simulink model "RM3old"  (R2018b)
settings: Solver=ode4  StartTime=0  StopTime=72.5  FixedStep=0.001  MaxStep=0.001  RelTol=1e-3  EnableMultiTasking=on
undefined symbols (not defined in the file or in its folder): body, constraint, pto
libraries: WECSim_Lib x5
settings Model: Creator=mlawson  LastModifiedBy=David
settings SolverCC: ZeroCrossControl=DisableAll  AlgebraicLoopSolver=LineSearch  AutoInsertRateTranBlk=on
settings DataIOCC: SaveFormat=Array  SaveOutput=off  SaveTime=off
settings OptimizationCC: LifeSpan=inf  SimCompilerOptimization=on
settings DebuggingCC: UnderspecifiedInitializationDetection=Classic  MergeDetectMultiDrivingBlocksExec=none  SolverPrmCheckMsg=warning  AllowSymbolicDim=off  StateNameClashWarn=warning  SFUnexpectedBacktrackingDiag=warning  SFNoUnconditionalDefaultTransitionDiag=warning  SFExecutionAtInitializationDiag=none
settings HardwareCC: ProdBitPerPointer=32  ProdBitPerSizeT=32  ProdBitPerPtrDiffT=32  ProdLargestAtomicFloat=None  ProdIntDivRoundTo=Undefined  ProdEndianess=Unspecified  ProdWordSize=32  ProdHWDeviceType=32-bit Generic
settings ModelReferenceCC: PropagateSignalLabelsOutOfModel=off
settings SFSimCC: SimUseLocalCustomCode=off
settings RTWCC: RTWUseLocalCustomCode=off
settings CodeAppCC: StateflowObjectComments=on
settings GRTTargetCC: TargetLangStandard=C89/C90 (ANSI)  GeneratePreprocessorConditionals=Disable all
settings ConfigComp: CovMetricSettings=dw  CovHtmlReporting=on  CovSaveCumulativeToWorkspaceVar=on  CovSaveSingleToWorkspaceVar=on  CovExternalEMLEnable=off  CovSFcnEnable=off
settings SimscapeCC: SimscapeNormalizeSystem=off
settings ConfigurationSet: Description=SimMechanics 2G
settings ExplorerConfigSet: InternalSimMechanicsExplorerSettings="<ExplorerConfiguration><canonicalview>default</canonicalview><TilePanel><TileInfo><Tiles Columns=\"1\" Count=\"1\" Rows=\"1\"><Column Left=\"2\" Weight=\"1\"/><Column Left=\"1335\"/><Row Top=\"2\" Weight=\"1\"/><Row Top=\"911\"/><Tile Height=\"1\" Width=\"1\" X=\"0\" Y=\"0\"/></Tiles></TileInfo><SceneInfo><SceneViewer><BGColor><R>0.60000002384185791</R><G>0.60000002384185791</G><B>0.60000002384185791</B></BGColor><Camera><Position><X>365.37645888990272</X><Y>-369.82486814446582</Y><Z>359.64809521743916</Z></Position><Center><X>-6.7351450971904585</X><Y>2.2867358426280204</Y><Z>-12.463508769654169</Z></Center><Up><X>-0.40824829046386307</X><Y>0.40824829046386307</Y><Z>0.81649658092772615</Z></Up><Left>-57.820127362122818</Left><Right>57.820127362122818</Right><Bottom>-38.308817187253304</Bottom><Top>38.308817187253304</Top></Camera></SceneViewer></SceneInfo></TilePanel></ExplorerConfiguration>"

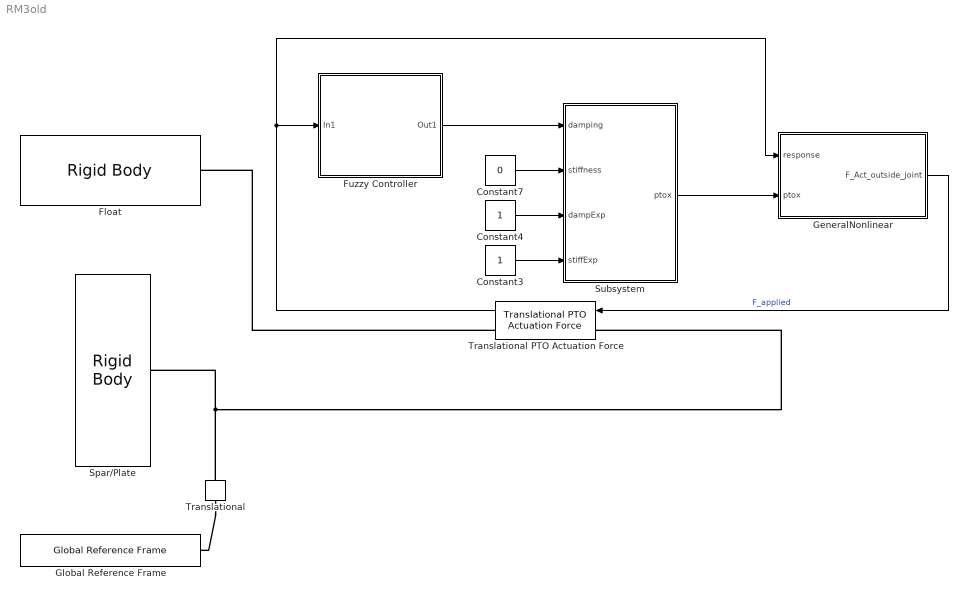
== system RM3old ==
  Constant3 : Constant
  Constant4 : Constant
  Constant7 : Constant  Value=0
  Float : WECSim_Lib/Body Elements/Rigid Body  body=body(1)
      settings: AttributesFormatString=%<body>  SourceProductName=WEC-Sim
  Fuzzy Controller : Subsystem
  GeneralNonlinear : Subsystem
  Global Reference Frame : WECSim_Lib/Frames/Global Reference Frame  waves=waves  simu=simu
      settings: SourceProductName=WEC-Sim
  Spar/Plate : WECSim_Lib/Body Elements/Rigid Body  body=body(2)
      settings: AttributesFormatString=%<body>  SourceProductName=WEC-Sim
  Subsystem : Subsystem
  Translational : WECSim_Lib/Constraints/Translational  constraint=constraint(1)
      settings: AttributesFormatString=%<constraint>  SourceProductName=WEC-Sim
  Translational PTO Actuation Force : WECSim_Lib/PTOs/Translational PTO Actuation Force  pto=pto(1)
      settings: AttributesFormatString=%<pto>  SourceProductName=WEC-Sim
  wires:
  GeneralNonlinear/1(F_Act_outside_joint) -> Translational PTO Actuation Force/1  "F_applied"
  Constant7/1 -> Subsystem/2(stiffness)
  Subsystem/1(ptox) -> GeneralNonlinear/2(ptox)
  Constant3/1 -> Subsystem/4(stiffExp)
  Translational PTO Actuation Force/1 -> GeneralNonlinear/1(response), Fuzzy Controller/1(In1)
  Constant4/1 -> Subsystem/3(dampExp)
  Fuzzy Controller/1(Out1) -> Subsystem/1(damping)
  connections:
  Translational/LConn1 -- Global Reference Frame/RConn1
  Translational/RConn1 -- Spar/Plate/RConn1 -- Translational PTO Actuation Force/LConn1
  Translational PTO Actuation Force/RConn1 -- Float/RConn1

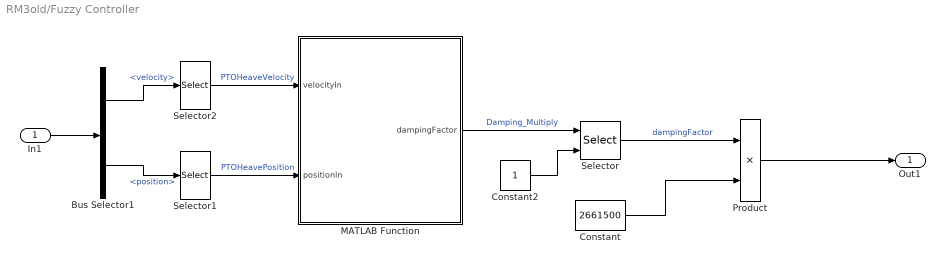
== system RM3old/Fuzzy Controller ==
  In1 : Inport
  Bus Selector1 : BusSelector  OutputSignals=velocity,position
  Constant : Constant  Value=2661500
  Constant2 : Constant
  MATLAB Function : MATLAB Function  TreatAsAtomicUnit=on  SystemSampleTime=0.01
  Product : Product
  Selector : Selector  InputPortWidth=2  IndexOptions=Index vector (port)  Indices=1  OutputSizes=1
  Selector1 : Selector  InputPortWidth=6  IndexOptions=Index vector (dialog)  Indices=3  OutputSizes=1
  Selector2 : Selector  InputPortWidth=6  IndexOptions=Index vector (dialog)  Indices=3  OutputSizes=1
  Out1 : Outport
  wires:
  Bus Selector1/2 -> Selector1/1  "<position>"
  Constant2/1 -> Selector/2
  Selector2/1 -> MATLAB Function/1(velocityIn)  "PTOHeaveVelocity"
  Bus Selector1/1 -> Selector2/1  "<velocity>"
  In1/1 -> Bus Selector1/1
  Selector1/1 -> MATLAB Function/2(positionIn)  "PTOHeavePosition"
  Selector/1 -> Product/1  "dampingFactor"
  Constant/1 -> Product/2
  MATLAB Function/1(dampingFactor) -> Selector/1  "Damping_Multiply"
  Product/1 -> Out1/1

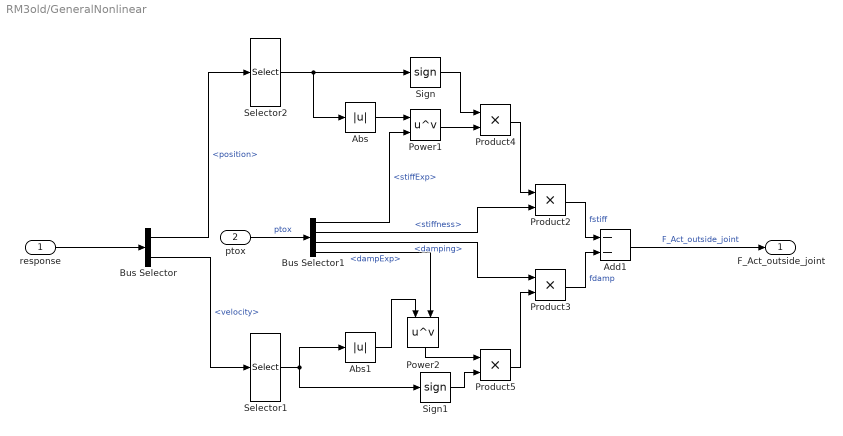
== system RM3old/GeneralNonlinear ==
  response : Inport
  ptox : Inport  Port=2
  Abs : Abs
  Abs1 : Abs
  Add1 : Sum  Inputs=--
  Bus Selector : BusSelector  OutputSignals=position,velocity
  Bus Selector1 : BusSelector  OutputSignals=stiffExp,stiffness,damping,dampExp
  Power1 : Math  Operator=pow  SaturateOnIntegerOverflow=on
  Power2 : Math  Operator=pow  SaturateOnIntegerOverflow=on
  Product2 : Product  Inputs=**
  Product3 : Product  Inputs=**
  Product4 : Product
  Product5 : Product
  Selector1 : Selector  InputPortWidth=6  IndexOptions=Index vector (dialog)  Indices=3  OutputSizes=1
  Selector2 : Selector  InputPortWidth=6  IndexOptions=Index vector (dialog)  Indices=3  OutputSizes=1
  Sign : Signum
  Sign1 : Signum
  F_Act_outside_joint : Outport
  wires:
  Power2/1 -> Product5/1
  Product5/1 -> Product3/2
  Sign/1 -> Product4/1
  Bus Selector1/3 -> Product3/1  "<damping>"
  Product2/1 -> Add1/1  "fstiff"
  response/1 -> Bus Selector/1
  Bus Selector1/1 -> Power1/2  "<stiffExp>"
  Bus Selector/2 -> Selector1/1  "<velocity>"
  Selector2/1 -> Sign/1, Abs/1
  Product4/1 -> Product2/1
  Add1/1 -> F_Act_outside_joint/1  "F_Act_outside_joint"
  Abs1/1 -> Power2/1
  Product3/1 -> Add1/2  "fdamp"
  Sign1/1 -> Product5/2
  Bus Selector1/2 -> Product2/2  "<stiffness>"
  Selector1/1 -> Abs1/1, Sign1/1
  Power1/1 -> Product4/2
  Bus Selector/1 -> Selector2/1  "<position>"
  Abs/1 -> Power1/1
  ptox/1 -> Bus Selector1/1  "ptox"
  Bus Selector1/4 -> Power2/2  "<dampExp>"

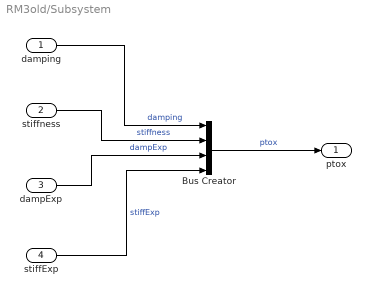
== system RM3old/Subsystem ==
  damping : Inport
  stiffness : Inport  Port=2
  dampExp : Inport  Port=3
  stiffExp : Inport  Port=4
  Bus Creator : BusCreator  Inputs=4
  ptox : Outport
  wires:
  stiffness/1 -> Bus Creator/2  "stiffness"
  stiffExp/1 -> Bus Creator/4  "stiffExp"
  Bus Creator/1 -> ptox/1  "ptox"
  damping/1 -> Bus Creator/1  "damping"
  dampExp/1 -> Bus Creator/3  "dampExp"

== matlab function RM3old/Fuzzy Controller/MATLAB Function ==
  data: velocityIn input; positionIn input; dampingFactor output size=[1 2]
function dampingFactor =...
    fuzzyLogicController(velocityIn, positionIn)
% Function to create and evaluate a fuzzy logic controller
% which implements a protection system for RM3 to limit relative movement
% between the float and spar, shedding power in the event of too-high wave conditions. The
% PTO implements an optimally linear damped control when within the travel limits,
% and applies a multiplication factor to the damping if the float is close
% to traveling out of bounds

% The functions and structures here are intended to be used as tools for the 
% general application of fuzzy logic controllers to wave energy converters.
% While not as complete as the MATLAB Fuzzy Logic Toolbox, this open source
% framework can be adapted to systems with an arbitrary number of inputs,
% outputs and rules, and can easily be expanded to include more membership
% function types, Fuzzy Operators, implication and aggregation methods, and
% defuzzification rules.

%%%%%%%%%%%%%%%%%%%%%%%%%%%%%%%%%%%%%%%
%% Define input membership functions %%
%%%%%%%%%%%%%%%%%%%%%%%%%%%%%%%%%%%%%%%
% Input membership function structures have the following expected fields:
% type -
% definingPoints -
% percentTrue -

%%% Velocity Input %%%
% Too fast Negative Velocity Limit
velocity.MFs.fastNeg.type = 'down step';
begin = -0.3146; finish = 0;
velocity.MFs.fastNeg.definingPoints = [begin finish];
velocity.MFs.fastNeg.percentTrue = NaN;

% Too Fast Positive Velocity
velocity.MFs.fastPos.type = 'step';
begin = 0.3146; finish = 1;
velocity.MFs.fastPos.definingPoints = [begin finish];
velocity.MFs.fastPos.percentTrue = NaN;

%%% Position Input %%%
% Too Negative Position Limit
position.MFs.low.type = 'down step';
begin = -0.5; finish = -0.4;
position.MFs.low.definingPoints = [begin finish];
position.MFs.low.percentTrue = NaN;

% In spec position
position.MFs.middle.type = 'trap';
begin = -0.5; asc = -0.4; dec = 0.4; finish = 0.5;
position.MFs.middle.definingPoints = [begin asc dec finish];
position.MFs.middle.percentTrue = NaN;

% Too Positive Position
position.MFs.high.type = 'step';
begin = 0.4; finish = 0.5;
position.MFs.high.definingPoints = [begin finish];
position.MFs.high.percentTrue = NaN;

%%%%%%%%%%%%%%%%%%%%
%% Fuzzify Inputs %%
%%%%%%%%%%%%%%%%%%%%
% pass input values to membership functions and update struct with
% membership truth values

position.MFs = fuzzifyInputs(positionIn, position.MFs);
velocity.MFs = fuzzifyInputs(velocityIn, velocity.MFs);

% organize all inputs into a single structure
inputs.position = position;
inputs.velocity = velocity;

%%%%%%%%%%%%%%%%%%%%%%%%%%%
%% Apply Fuzzy Operators %%
%%%%%%%%%%%%%%%%%%%%%%%%%%%
% Define Rule antecedents and apply fuzzy operators to multi-input rules

% Rule 1 antecedent: If velocity is fast positive and position is high
ruleOneInputMFs = [inputs.velocity.MFs.fastPos.percentTrue  inputs.position.MFs.high.percentTrue];
ruleOneAntecedent = applyFuzzyOperator(ruleOneInputMFs, 'minAnd');

% Rule 2 antecedent: If position is middle
% Sinlge input rule does not require fuzzy operator
ruleTwoInputMF = [position.MFs.middle.percentTrue];
ruleTwoAntecedent = ruleTwoInputMF;

% Rule 3 antecedent: If velocity is fast negative and position is low
ruleThreeInputMFs = [inputs.velocity.MFs.fastNeg.percentTrue  position.MFs.low.percentTrue];
ruleThreeAntecedent = applyFuzzyOperator(ruleThreeInputMFs, 'minAnd');

%%%%%%%%%%%%%%%%%%%%%%%%%%%%
%% Apply Rule Implication %%
%%%%%%%%%%%%%%%%%%%%%%%%%%%%

% Specify membership functions for outputs and Generate Consequent Membership Functions

% Rule 1: If velocity is fast positive and position is high damping is
% overdamped

% Overdamped Membership Function for multiplier
overDamped.type = 'triangle';
begin = 1; peak = 40; finish = 41;
overDamped.definingPoints = [begin peak finish];


% Rule 3: If velocity is fast positive and position is high damping is
% overdamped



% Rule 2:  If position is middle damping is optimal
% Base Membership Function
optimal.type = 'triangle';
begin = 0; peak = 1; finish = 40;
optimal.definingPoints = [begin peak finish];


% Consequent Membership Functions
ruleOne = applyImplicationMethod(ruleOneAntecedent,overDamped,'min');
ruleTwo = applyImplicationMethod(ruleTwoAntecedent,optimal,'min');
ruleThree = applyImplicationMethod(ruleThreeAntecedent,overDamped,'min');

% organize by: outputs -> fuzzy sets -> rules
% Each output struct expects a CMF field containing the fuzzy sets which
% belong to that output and a range field containing the limits of the
% output
% Each output fuzzy set struct expects a aggregation type for rules which apply
% and a rules struct containing the modified MF for those rules which apply

dampingMultiplier.baseMFs.overDamped = overDamped;
dampingMultiplier.CMFs.overDamped.ruleAggregation = 'max';
dampingMultiplier.CMFs.overDamped.rules.ruleOne = ruleOne;
dampingMultiplier.CMFs.overDamped.rules.ruleThree = ruleThree;

dampingMultiplier.baseMFs.optimal = optimal;
dampingMultiplier.CMFs.optimal.rules.ruleTwo = ruleTwo;

% use NaN for no limit
dampingMultiplier.range = [1 40];

%%%%%%%%%%%%%%%%%%%%%
%% Aggregate Rules %%
%%%%%%%%%%%%%%%%%%%%%
% expected aggregation methods - 
outputs.dampingMultiplier = dampingMultiplier;
outputs.dampingMultiplier.aggregatedFunction = aggregateCMFs(dampingMultiplier, 'sum');

%%%%%%%%%%%%%%%%%%%%%%%%%%
%% Defuzzify output MFs %%
%%%%%%%%%%%%%%%%%%%%%%%%%%
% Defuzzify final output membership functions and assign crisp values
% expected defuzzification methods: centroid, bisector, mean of maxima (MOM),
% largest of maxima (LOM), smallest of maxima (SOM)

 dampingFactor = defuzzify(outputs.dampingMultiplier, 'MOM');

end
%%%%%%%%%%%%%%%%%%
%% End of Main %%
%%%%%%%%%%%%%%%%%%
% begin functions


function fuzzufiedInput = fuzzifyInputs(inValue, MFs)
% Function to fuzzify crisp input variables
% inputs: 
%   invalue - crisp input value
%   MFs - struct of fuzzy set membership functions for an input
% outputs: 
%   fuzzufiedInput - updated MFs struct with fuzzy truth value for each MF

    % list of memberships for this input
    listMFs = fieldnames(MFs);

    % go through each membership function
    for k=1:numel(listMFs)
        thisMF = MFs.(listMFs{k});

        mfType = thisMF.type;

        %calculate its percentTrue strength based on type
        switch mfType
            case 'triangle'
                MFs.(listMFs{k}).percentTrue = tri_MF(inValue,...
                    MFs.(listMFs{k}).definingPoints(1), MFs.(listMFs{k}).definingPoints(2), MFs.(listMFs{k}).definingPoints(3), 1);
            case 'step'
                MFs.(listMFs{k}).percentTrue = open_trap_right(inValue,...
                     MFs.(listMFs{k}).definingPoints(1), MFs.(listMFs{k}).definingPoints(2), 1);
            case 'down step'
                 MFs.(listMFs{k}).percentTrue = open_trap_left(inValue,...
                     MFs.(listMFs{k}).definingPoints(1), MFs.(listMFs{k}).definingPoints(2), 1);
            case 'trap'
                 MFs.(listMFs{k}).percentTrue = trap(inValue,...
                     MFs.(listMFs{k}).definingPoints(1), MFs.(listMFs{k}).definingPoints(2), MFs.(listMFs{k}).definingPoints(3), MFs.(listMFs{k}).definingPoints(4), 1);
            otherwise
                disp('membership function type not defined');
        end
    end

    fuzzufiedInput = MFs;

end

function membership = tri_MF(inValue, begin, peak, finish, maxTruth)
% Evaluate input according to triangular MF
% inputs: 
%   inValue - system input value 
%   begin - input value triangle begins to rise, before which truth value is 0
%   peak - input value triangle peaks and begins to fall
%   finish - input value triangle returns to 0, after which which truth value is 0
%   maxTruth - truth value for peak input, default 1 for input MFs
% outputs:
%   membership - truth value between 0 and 1 corresponding to the input    
%
    if inValue < peak
        if inValue <= begin
            membership = 0;
        else
            membership = (maxTruth/(peak - begin)) * (inValue-peak) + maxTruth;
        end
    elseif inValue > peak
        if inValue >= finish
            membership = 0;
        else
            membership = ((-1*maxTruth)/(finish - peak)) * (inValue-peak) + maxTruth;
        end
    else
        membership = maxTruth;
    end
end

function membership = open_trap_left(inValue, begin, finish, maxTruth)
% Evaluate input according to falling step membership function
% inputs: 
%   inValue - system input value 
%   begin - input value step begins to fall, before which truth value is 1
%   finish - input value trap reaches 0, after which which truth value is 0
%   maxTruth - truth value for input below 'begin', default 1 for input MFs
% outputs:
%   membership - truth value between 0 and 1 corresponding to the input    
%
    if inValue < begin
        membership = maxTruth;
    elseif inValue > finish
        membership = 0;
    else
        membership = (maxTruth/(begin - finish))*(inValue - begin) + maxTruth;
    end
end

function membership = open_trap_right(inValue, begin, finish, maxTruth)
% Evaluate input according to rising step membership function
% inputs: 
%   inValue - system input value 
%   begin - input value step begins to rise, before which truth value is 0
%   finish - input value trap reaches 1, after which which truth value is 1
%   maxTruth - truth value for input above 'finish', default 1 for input MFs
% outputs:
%   membership - truth value between 0 and 1 corresponding to the input   

    if inValue < begin
        membership = 0;
    elseif inValue > finish
        membership = maxTruth;
    else
        membership = (maxTruth/(finish - begin))*(inValue - finish) + maxTruth;
    end
end

function membership = trap(inValue, begin, asc, dec, finish, maxTruth)
% Evaluate input according to trapezoidal MF
% inputs: 
%   inValue - system input value 
%   begin - input value at which trapezoid begins to rise, before which truth value is 0
%   asc - input value at which trapezoid reaches plateau value
%   dec - input value at which trapezoid returns to 0, after which truth value is 0
%   maxTruth - truth value for plateau inputs, default 1 for input MFs
% outputs:
%   membership - truth value between 0 and 1 corresponding to the input    
%
    if ( inValue < begin ) || ( inValue > finish )
        membership = 0;
    elseif inValue < asc
        membership = (maxTruth/(asc-begin))*(inValue - begin);
    elseif inValue > dec
        membership = (maxTruth/(dec-finish))*(inValue - finish);
    else
        membership = maxTruth;
    end
end


function antecedentTruth = applyFuzzyOperator(inputMembershipTruth, fuzzyOperator)
% applies a fuzzy operator to produce a single 
% antecedent value for multi-input fuzzy rules
% Inputs: 
%       inputMembershipTruth - vector of analog truth values for
%       input membership function values relevant to rule
%       fuzzyOperator - Fuzzy operator to select a single truth value for the
%       antecedent of the rule
    switch fuzzyOperator
        case 'minAnd'
            antecedentTruth = min(inputMembershipTruth);
        case 'prodAnd'
            antecedentTruth = prod(inputMembershipTruth);
        case 'maxOr'
            antecedentTruth = max(inputMembershipTruth);
        case 'average'
            antecedentTruth = mean(inputMembershipTruth);
        otherwise
            disp('Specified Fuzzy Operator is not defined');
    end
end

function consequentMF = applyImplicationMethod(antecedent, outputMembership, implicationMethod)
% function to implicate rules
% inputs:
%   antecedent - single truth value for the rule's antecedent
%   outputMembership - membership funciton structure for output
%   implicationMethod - an implication method
% outputs: 
%   consequentMF - membership function shaped by the antecedent
    if (antecedent == 1) || (antecedent == 0) || strcmp(implicationMethod,'prod')
        outCopy = outputMembership;
        outCopy.maxVal = antecedent;
        consequentMF = outCopy;
    elseif strcmp(implicationMethod,'min')
        switch outputMembership.type
            case 'trap'
                outTrap = outputMembership;
                outTrap.maxVal = antecedent;
                outTrap.definingPoints(2) = antecedent * (outputMembership.definingPoints(2) - outputMembership.definingPoints(1)) + outputMembership.definingPoints(1);
                outTrap.definingPoints(3) = antecedent * (outputMembership.definingPoints(3) - outputMembership.definingPoints(4)) + outputMembership.definingPoints(4);
                consequentMF = outTrap;
            case 'step'
                outStep = outputMembership;
                outStep.maxVal = antecedent;
                outStep.definingPoints(2) = antecedent * (outputMembership.definingPoints(2) - outputMembership.definingPoints(1)) + outputMembership.definingPoints(1);
                consequentMF = outStep;
            case 'down step'
                outDownStep = outputMembership;
                outDownStep.definingPoints(1) = antecedent * (outputMembership.definingPoints(1) - outputMembership.definingPoints(2)) + outputMembership.definingPoints(2);
                outDownStep.maxVal = antecedent;
                consequentMF = outDownStep;
            case 'triangle' % Chop the top off
                outTri.type = 'trap';
                outTri.definingPoints = zeros(1,4);
                outTri.definingPoints(1) = outputMembership.definingPoints(1);
                outTri.definingPoints(4) = outputMembership.definingPoints(3);
                outTri.definingPoints(2) = antecedent * (outputMembership.definingPoints(2) - outputMembership.definingPoints(1)) + outputMembership.definingPoints(1);
                outTri.definingPoints(3) = antecedent * (outputMembership.definingPoints(2) - outputMembership.definingPoints(3)) + outputMembership.definingPoints(3);
                outTri.maxVal = antecedent;
                consequentMF = outTri;
            otherwise
                disp('membership function specified for output not defined');
        end
    else
        disp('Specified implication method is not defined');
        consequentMF = 0;
    end
end

function mfTruth = evalMF(inValue, MF)
% General function to evaluate membership functions may not have a max of 1
% inputs:
%   inValue - value to evaluate membership for
%   MF - membership function struct which expects a maxVal field
% outputs:
%   single truth value
%

mfType = MF.type;
        %calculate its percentTrue strength based on
        switch mfType
            case 'triangle'
                mfTruth = tri_MF(inValue,...
                    MF.definingPoints(1), MF.definingPoints(2), MF.definingPoints(3),  MF.maxVal);
            case 'step'
                mfTruth = open_trap_right(inValue,...
                     MF.definingPoints(1), MF.definingPoints(2), MF.maxVal);
            case 'down step'
                 mfTruth = open_trap_left(inValue,...
                     MF.definingPoints(1), MF.definingPoints(2), MF.maxVal);
            case 'trap'
                 mfTruth = trap(inValue,...
                     MF.definingPoints(1), MF.definingPoints(2), MF.definingPoints(3), MF.definingPoints(4), MF.maxVal);
            otherwise
                mfTruth = NaN;
                disp('membership function type not defined');
        end
end

function singleTruthFunction = performAgg(truthMatrix, aggregationMethod)
% function to aggreate rules
% inputs:
%   truthMatrix: matrix where each row represents the truth value of the
%   corresponding rule's membership function, evaluated at the necessary
%   points to get a complete detailed aggregation
%

    switch aggregationMethod
        case 'max'
            singleTruthFunction = max(truthMatrix,[],1);
        case 'min'
            singleTruthFunction = min(truthMatrix,[],1);
        case 'mean'
            singleTruthFunction = mean(truthMatrix,[],1);
        case 'prod'
            singleTruthFunction = truthMatrix(1,:)
            for r = 2:length(truthMatrix(:,1))
                singleTruthFunction = truthMatrix(r,:).*singleTruthFunction;
            end
        case 'sum'
            singleTruthFunction = truthMatrix(1,:);
            if length(truthMatrix(:,1)) > 1
                for r = 2:length(truthMatrix(:,1))
                    singleTruthFunction = truthMatrix(r,:) + singleTruthFunction;
                end
            end
        otherwise
            disp('specified aggregation method not defined');
    end
end

function aggregatedMF = aggregateCMFs(outputName, aggregationMethod)
% function to aggregate all rules' MFs which apply to an output fuzzy set,
% then to aggregate all sets which apply to the output
% inputs: 
%   outputName - structure containing the fuzzy sets for each input, and
%   consequent membership functions for each rule of each set
%   aggregationMethod - an aggregation method for the sets
% outputs:
%   aggregatedMF - 2 row vector representing the final aggregated membership 
%   function for the output with the first row being the output values (x
%   axis) and the second row as the corresponding truth value (y axis)

listStates = fieldnames(outputName.CMFs);
outMin = outputName.range(1);
outMax = outputName.range(2);

% Loop 1 to aggregate rules for each state/MF (e.g. rule 2 and 3 both affect
% overdamped set, their consequent MF must be combined)
for p=1:numel(listStates)
    thisCMF = outputName.CMFs.(listStates{p});
    
    listRules = fieldnames(thisCMF.rules);
    if numel(listRules) > 1
        if (thisCMF.ruleAggregation)
            ruleAgg = thisCMF.ruleAggregation;
        else
            disp('If multiple rules affect a member function a rule aggregation must be specified');
        end
    end
    
    % get unique list of defining points for this state (from all rules for
    % this state)

    % first loop to get the length of all defining points for this state for
    % preallocation purposes
    ruleRangeMaxLength = 0;
    for s=1:numel(listRules)
        thesePoints = outputName.CMFs.(listStates{p}).rules.(listRules{s}).definingPoints;
        ruleRangeMaxLength = ruleRangeMaxLength + numel(thesePoints);
    end
    
    %Now assign all points to range vector
    fullRuleRange = NaN(1,ruleRangeMaxLength);
    fullRuleRangeIndex=1;
    for s=1:numel(listRules)
        thesePoints = outputName.CMFs.(listStates{p}).rules.(listRules{s}).definingPoints;
        for t = 1:numel(thesePoints)
            fullRuleRange(fullRuleRangeIndex) = thesePoints(t);
            fullRuleRangeIndex = fullRuleRangeIndex+1;
        end
        
    end
    
    % remove duplicates
    uniqueRuleRange = unique(fullRuleRange(~isnan(fullRuleRange)));

    
    % loop through comparing each rule and add any rule intersections to
    % the list of defining points
    
    % first count the max number of points the intersections could add, for
    % allocation purposes
    ruleIntersectionsMaxLength = 0;
    for s=1:numel(listRules)
        compareRuleOne = thisCMF.rules.(listRules{s});
        
        for t = (s+1):numel(listRules)
            compareRuleTwo = thisCMF.rules.(listRules{t});
            
            ruleOneTruth = NaN(1,numel(uniqueRuleRange));
            ruleTwoTruth = NaN(1,numel(uniqueRuleRange));
            
            % create y values for each rule MF
            for m = 1:numel(uniqueRuleRange)
               uniqueRuleRange(m);
               ruleOneTruth(m) = evalMF(uniqueRuleRange(m),compareRuleOne);
               ruleTwoTruth(m) = evalMF(uniqueRuleRange(m),compareRuleTwo);
            end
            
            ruleX = MFintersect(uniqueRuleRange, ruleOneTruth, ruleTwoTruth);
            ruleIntersectionsMaxLength = ruleIntersectionsMaxLength + numel(ruleX);
        end
    end
    
    % preallocate
    rangeWithIntersections = NaN(1,numel(ruleIntersectionsMaxLength));
    
    % Now go through and assign
    intersectionIndex = 1;
    for s=1:numel(listRules)
        compareRuleOne = thisCMF.rules.(listRules{s});
        
        for t = (s+1):numel(listRules)
            compareRuleTwo = thisCMF.rules.(listRules{t});
            
            ruleOneTruth = NaN(1,numel(uniqueRuleRange));
            ruleTwoTruth = NaN(1,numel(uniqueRuleRange));
            
            % create y values for each rule MF
            for m = 1:numel(uniqueRuleRange)
               uniqueRuleRange(m);
               ruleOneTruth(m) = evalMF(uniqueRuleRange(m),compareRuleOne);
               ruleTwoTruth(m) = evalMF(uniqueRuleRange(m),compareRuleTwo);
            end
            
            ruleX = MFintersect(uniqueRuleRange, ruleOneTruth, ruleTwoTruth);
            ruleIntersections = ruleX;
            for n = 1:numel(ruleIntersections(1,:))
                rangeWithIntersections(intersectionIndex) = ruleIntersections(1,n);
                intersectionIndex = intersectionIndex + 1;
            end
        end
    end
    
    % remove duplicates
    uniqueRangeIntersections = unique(rangeWithIntersections);
    
    % combine the two and remove any lingering NaN
    finalOutRange = [uniqueRangeIntersections  uniqueRuleRange];
    uniqueFinalRange = unique(finalOutRange(~isnan(finalOutRange)));
 
    % Now we have the list of output values which define the corners and
    % possible intersections of all rules for this MF state. Define a
    % matrix where each row will be a rule MF for aggregation for all
    % points along the relevant range
    
    stateRulesMat = zeros(numel(listRules),numel(uniqueFinalRange));
    
    for row=1:numel(listRules)
        thisRule = thisCMF.rules.(listRules{row});
        for col = 1:numel(uniqueFinalRange)
            stateRulesMat(row,col) = evalMF(uniqueFinalRange(col),thisRule);
        end
    end
    
    % Finally can aggregate rules without losing any MF resolution
    outVari.(listStates{p}).func = [uniqueFinalRange; performAgg(stateRulesMat, aggregationMethod)];
        
end

% Now aggregate all the set MFs (e.g. overdamped and optimal)


stateList = fieldnames(outVari);

% this loop get all the X over each state MF
% first loop that counts for preallocate
maxDefiningPointsCount = 0;
for p = 1:numel(stateList)
    thisState = outVari.(stateList{p});
    maxDefiningPointsCount = maxDefiningPointsCount + numel(thisState.func(1,:));
end

% preallocate
outRange = NaN(1,maxDefiningPointsCount);
outRangeIndex = 1;

% second loop assigns
for p = 1:numel(stateList)
    thisState = outVari.(stateList{p});

    for q = 1:numel(thisState.func(1,:))
        outRange(outRangeIndex) = thisState.func(1,q);
        outRangeIndex = outRangeIndex + 1;
    end
    
end

outRangeLimits = [outRange outMin outMax];


uniqueOutRange = unique(outRangeLimits);

stateOutMat = zeros(numel(stateList),numel(uniqueOutRange));
for row = 1:numel(stateList)
    thisFuncX = outVari.(stateList{row}).func(1,:);
    thisFuncT = outVari.(stateList{row}).func(2,:);
    for col = 1:numel(uniqueOutRange)
        if (uniqueOutRange(col) > max(thisFuncX)) || (uniqueOutRange(col) < min(thisFuncX))
            stateOutMat(row,col) = interp1(thisFuncX,thisFuncT,uniqueOutRange(col),'nearest','extrap');
        else
            stateOutMat(row,col) = interp1(thisFuncX,thisFuncT,uniqueOutRange(col),'linear');
        end
    end
end

% TODO: I'm going to need the x values of intersections here too...?

% loop through rows of stateOutMat vs unique out range to count intersections
maxSetIntersects = 0;
[numSetRows ~] = size(stateOutMat);
for s = 1:numSetRows
    setCompareOne = stateOutMat(s,:);
    
    for t = s+1:numSetRows
        setCompareTwo = stateOutMat(t,:);
        
        setX = MFintersect(uniqueOutRange, setCompareOne, setCompareTwo);
        maxSetIntersects = maxSetIntersects + numel(setX);
        
    end
end

% preallocate
setIntersectionX = NaN(1,maxSetIntersects);
intersectionCount = 1;

% loop to assign them
for s = 1:numSetRows
    setCompareOne = stateOutMat(s,:);
    
    for t = s+1:numSetRows
        setCompareTwo = stateOutMat(t,:);
        
        setX = MFintersect(uniqueOutRange, setCompareOne, setCompareTwo);
        
        for u = 1:numel(setX(1,:))
            setIntersectionX(intersectionCount) = setX(1,u);
            intersectionCount = intersectionCount + 1;
        end
        
    end
end

% add them to range
finalOutRangeWithIntersects = [uniqueOutRange setIntersectionX];
% removeNaNs and dups
finalRange = unique(finalOutRangeWithIntersects(~isnan(finalOutRangeWithIntersects)));

% re-create state out mat with new output range
finalStateOutMat = NaN(numel(stateList),numel(finalRange));
for row = 1:numel(stateList)
    thisFuncX = uniqueOutRange;
    thisFuncT = stateOutMat(row,:);
    
    for col = 1:numel(finalRange)
        if (finalRange(col) > max(thisFuncX)) || (finalRange(col) < min(thisFuncX))
            finalStateOutMat(row,col) = interp1(thisFuncX,thisFuncT,finalRange(col),'nearest','extrap');
        else
            finalStateOutMat(row,col) = interp1(thisFuncX,thisFuncT,finalRange(col),'linear');
        end
    end
end



%Finally, finally, finally can aggregate all output's set MFs without losing resolution
aggregatedFunction = performAgg(finalStateOutMat, aggregationMethod);

% return as a linear interpolate function
aggregatedMF = [finalRange; aggregatedFunction];

 end

function crisp = defuzzify(outputFun, defuzzificationMethod)
% function to call relevant defuzzification function

outMin = outputFun.range(1);
outMax = outputFun.range(2);

func = outputFun.aggregatedFunction;
switch defuzzificationMethod
    case 'centroid'
        crisp = getCentroidX(func);
    case 'bisector'
        crisp = bisectSearch(func,min(func(1,:)),max(func(1,:)));
    case 'LOM'
        crisp = maxima(func,'largest');
    case 'MOM'
        crisp = maxima(func,'mean');
    case 'SOM'
        crisp = maxima(func,'smallest');
    otherwise disp('Specified defuzzification method not defined');
        crisp = NaN;
end

% Keep it in range
if crisp > outMax && ~isNaN(outMax)
    crisp = outMax;
elseif crisp < outMin  && ~isNaN(outMin)
    crisp = outMin;
end

end

function centroX = getCentroidX(curve)
% function to return output value corresponding to MF centroid

    if curve(2,end) ~= 0
        polydCurve = [curve [curve(1, end) ; 0 ] ];
    else
         polydCurve = curve;
    end

    polyin = polyshape(ploydCurve','Simplify',true);
    polyin = simplify(polyin,'KeepCollinearPoints',false);
    [x,~] = centroid(polyin);    
    centroX = x;
end

function xBisect = bisectSearch(curve,searchMin,seaarchMax)
% function to return output value corresponding to MF bisector

    xBisect = 0;
    fullX = curve(1,:);
    fullY = curve(2,:);

    totalArea = trapz(fullX,fullY);
    
    midX = (searchMin + seaarchMax)/2;
    midY = interp1(fullX,fullY,midX,'linear');
    
    
    halfXTest = [fullX(fullX < midX) midX];
    halfYTestLen = numel(fullX(fullX < midX));
    halfYTest = [fullY(1:halfYTestLen) midY];
    halfAreaTest = trapz(halfXTest,halfYTest);
    
    if round(halfAreaTest,4) == round(0.5*totalArea,4)
        xBisect = midX;
    elseif halfAreaTest > 0.5*totalArea
        xBisect = bisectSearch(curve,searchMin,midX);
    elseif halfAreaTest < 0.5*totalArea
        xBisect = bisectSearch(curve,midX,seaarchMax);
    end
end

function aMax = maxima(curve,type)
% function to return output value corresponding to MF maxima type

aMax = 0;
fullX = curve(1,:);
fullY = curve(2,:);

% if there is a single most true point
if size(fullY(fullY == max(fullY))) == 1
    % return the x
    aMax = fullX(find(fullY==max(fullY)));
else
    switch type
        case 'largest'
            % largest = highest absolute value 
            maximaXs = fullX(find(fullY==max(fullY)));
            maximaXsMag = abs(maximaXs);
            
            if size(maximaXsMag(maximaXsMag == max(maximaXsMag))) == 1
                % if there's only 1, return the x
                aMax = maximaXs(find(maximaXsMag==max(maximaXsMag)));
            else
                % if there's a tie (i.e. the corresponding positive and
                % negative x are both the most true) return the negative
                % one
                aMax = maximaXs(find(maximaXs==-1*max(maximaXsMag)));
            end
        case 'mean'
            maximaXs = fullX(find(fullY==max(fullY)));
            aMax = (max(maximaXs) + min(maximaXs))/2;
            %if there are two separate max plateaus, should their average be
            %weighted?, like find the middle each plateaus, and take an average
            %of the MOMs weighted by their length?? too complicated
        case 'smallest'
            % smallest = lowest absolute value 
            maximaXs = fullX(find(fullY==max(fullY)));
            maximaXsMag = abs(maximaXs);
            
            if size(maximaXsMag(maximaXsMag == max(maximaXsMag))) == 1
                % if there's only 1, return the x
                aMax = maximaXs(find(maximaXsMag==max(maximaXsMag)));
            else
                % if there's a tie (i.e. the corresponding positive and
                % negative x are both the most true values) return the 
                % negative one
                aMax = maximaXs(find(maximaXs==-1*max(maximaXsMag)));
            end
    end

end

end

function intersectionsX = MFintersect(X, Y1, Y2)

% TODO: enforce X and Y's length

% get two consecutive sets of truth values. subtract them from each other,
% and compare the signs. if they're different, find the interesection

% if it does, solve the 2 linear equations for the intersection.

% count for pre-allocate
intersectionsCount = 0;
for i = 2:numel(X)
    if (sign(Y1(i-1)-Y2(i-1)) ~= sign(Y1(i)-Y2(i)))
        intersectionsCount = intersectionsCount + 1;
    end
end

% preallocate
intersectionsX = NaN(1,intersectionsCount);
intersectionNumber = 1;
    
for i = 2:numel(X)

    % check if who's on top changed
    if (sign(Y1(i-1)-Y2(i-1)) ~= sign(Y1(i)-Y2(i)))
        
        % line slopes in intersection interval
        M1 = (Y1(i-1)-Y1(i))/(X(i-1)-X(i));
        M2 = (Y2(i-1)-Y2(i))/(X(i-1)-X(i));
        
        % X value of intersection
        intersectionsX(intersectionNumber) = ...%find the x value of intersections
            X(i) + (Y2(i)-Y1(i))/(M1-M2);
        intersectionNumber = intersectionNumber + 1;
    end
    
    if intersectionNumber > intersectionsCount
        break;
    end
end    


end
